simulink model "FourModesSerial"  (R2022b)
settings: Solver=FixedStepAuto  StartTime=0.0  StopTime=10.0  FixedStep=1e-3  RelTol=1e-3  EnableMultiTasking=on
undefined symbols (not defined in the file): D0, D1, D10, D11, D12, D13, D2, D3, D4, D5, D6, D7, D8, D9, PTA0, PTA1, PTA2, PTB23, PTB9, PTC16, PTC17, PTC2, PTC3, PTC4, PTD0, PTD1, PTD2, PTD3
libraries: frdmk64flib x17, etargetslib x2, dspstat3 x1
settings Model: ExtModeTrigDuration=5  Creator=16475  LastModifiedBy=16475
settings OptimizationCC: EnhancedBackFolding=on  PassReuseOutputArgsAs=Individual arguments  ZeroExternalMemoryAtStartup=off  ZeroInternalMemoryAtStartup=off  MaxStackSize=64  OptimizeBlockOrder=speed  DifferentSizesBufferReuse=on  OptimizationCustomize=off  EfficientTunableParamExpr=on
settings DebuggingCC: ParameterTunabilityLossMsg=error
settings HardwareCC: ProdBitPerPointer=32  ProdBitPerSizeT=32  ProdBitPerPtrDiffT=32  ProdLargestAtomicInteger=Long  ProdLargestAtomicFloat=Double  ProdWordSize=32  ProdHWDeviceType=ARM Compatible->ARM Cortex
settings SFSimCC: MATLABDynamicMemAlloc=off
settings RTWCC: Description=Embedded Coder  SystemTargetFile=ert.tlc  HardwareBoard=NXP FRDM-K64F  TLCOptions="-aInlineSetEventsForThisBaseRateFcn=TLC_FALSE -aSuppressMultiTaskScheduler=TLC_FALSE  -aRateBasedStepFcn=0"  TemplateMakefile=ert_default_tmf  Toolchain=GNU Tools for ARM Embedded Processors
settings CodeAppCC: ForceParamTrailComments=on  IgnoreCustomStorageClasses=off  OperatorAnnotations=on  SimulinkDataObjDesc=on  SFDataObjDesc=on  InsertBlockDesc=on
settings ERTTargetCC: ExtModeTransport=4  ExtModeMexFile=sendToCommService

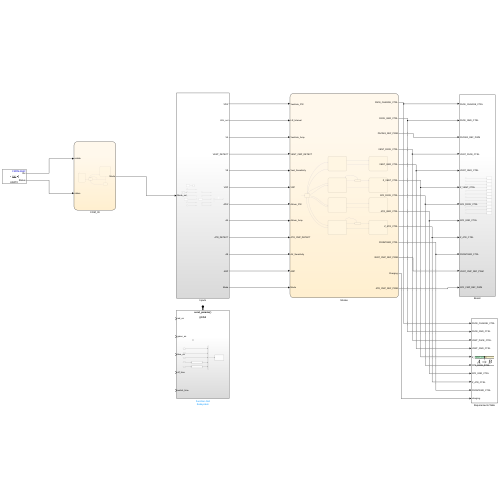
[thumbnail: Simulink's stored preview of the top-level diagram]
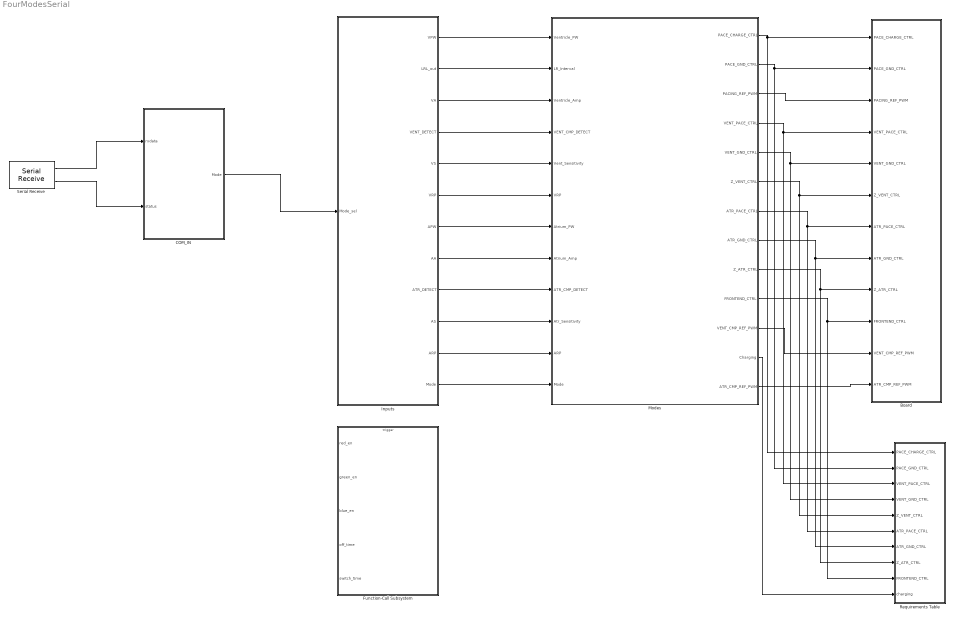
== system FourModesSerial ==
  Board : Subsystem
  COM_IN : Stateflow chart  TreatAsAtomicUnit=on
  Function-Call Subsystem : Subsystem  TreatAsAtomicUnit=on
  Inputs : Subsystem
  Modes : Stateflow chart  TreatAsAtomicUnit=on
      settings: PortSchema="{\"entries\":[{\"content\":{\"sides\":[{\"content\":{\"connectorIds\":[\"In1\",\"In2\",\"In3\",\"In4\",\"In5\",\"In6\",\"In7\",\"In8\",\"In9\",\"In10\",\"In11\",\"In12\"]},\"type\":\"ConnectorPlacement.EquallySpacedRectSide\",\"uuid\":\"a3e94f58-3093-42a5-91db-f56c9d127bee\"},{\"content\":{\"connectorIds\":[\"Out1\",\"Out2\",\"Out3\",\"Out5\",\"Out4\",\"Out7\",\"Out6\",\"Out8\",\"Out9\",\"Out10\",\"Out11\",\"Out12\",\"Out13\"],\"side\":\"RIGHT\"},\"type\":\"ConnectorPlacement.EquallySpacedRectSide\",\"uuid\":\"289ad049-9840-4721-af22-1385d5696f7c\"},{\"content\":{\"connectorIds\":[],\"side\":\"TOP\"},\"type\":\"ConnectorPlacement.EquallySpacedRectSide\",\"uuid\":\"4602f2ad-cb91-4c7a-9db6-6571445db01f\"}]},\"type\":\"ConnectorPlacement.EquallySpacedConnector\",\"uuid\":\"bfd50937-4990-4c1b-ba87-ff4dc7d3240f\"}],\"packageUris\":[\"http://schema.mathworks.com/mf0/Connector/R2020b\"],\"version\":\"1.0\"}"
  Requirements Table : Requirements Table  TreatAsAtomicUnit=on
  Serial Receive : frdmk64flib/Serial Receive  SCIModule=0  Baudrate=uint32(9600)  Parity=None  StopBits=1  HardwareFlowControl=None  ByteOrder=LittleEndian  DataType=uint8  DataLength=11  BlockingMode=off  OutputStatus=on  SampleTime=-1
  wires:
  Modes/11(VENT_CMP_REF_PWM) -> Board/11(VENT_CMP_REF_PWM)
  Modes/1(PACE_CHARGE_CTRL) -> Requirements Table/1(PACE_CHARGE_CTRL), Board/1(PACE_CHARGE_CTRL)
  Modes/2(PACE_GND_CTRL) -> Requirements Table/2(PACE_GND_CTRL), Board/2(PACE_GND_CTRL)
  Modes/3(PACING_REF_PWM) -> Board/3(PACING_REF_PWM)
  Modes/5(VENT_PACE_CTRL) -> Requirements Table/3(VENT_PACE_CTRL), Board/4(VENT_PACE_CTRL)
  Modes/4(VENT_GND_CTRL) -> Requirements Table/4(VENT_GND_CTRL), Board/5(VENT_GND_CTRL)
  Modes/7(Z_VENT_CTRL) -> Requirements Table/5(Z_VENT_CTRL), Board/6(Z_VENT_CTRL)
  Modes/6(ATR_PACE_CTRL) -> Requirements Table/6(ATR_PACE_CTRL), Board/7(ATR_PACE_CTRL)
  Modes/8(ATR_GND_CTRL) -> Requirements Table/7(ATR_GND_CTRL), Board/8(ATR_GND_CTRL)
  Modes/9(Z_ATR_CTRL) -> Requirements Table/8(Z_ATR_CTRL), Board/9(Z_ATR_CTRL)
  Modes/10(FRONTEND_CTRL) -> Requirements Table/9(FRONTEND_CTRL), Board/10(FRONTEND_CTRL)
  Modes/12(Charging) -> Requirements Table/10(charging)
  Inputs/1(VPW) -> Modes/1(Ventricle_PW)
  Inputs/2(LRL_out) -> Modes/2(LR_Interval)
  Inputs/3(VA) -> Modes/3(Ventricle_Amp)
  Inputs/4(VENT_DETECT) -> Modes/4(VENT_CMP_DETECT)
  Inputs/5(VS) -> Modes/5(Vent_Sensitivity)
  Inputs/6(VRP) -> Modes/6(VRP)
  Inputs/7(APW) -> Modes/7(Atrium_PW)
  Inputs/8(AA) -> Modes/8(Atrium_Amp)
  Inputs/9(ATR_DETECT) -> Modes/9(ATR_CMP_DETECT)
  Inputs/10(AS) -> Modes/10(Atr_Sensitivity)
  Inputs/11(ARP) -> Modes/11(ARP)
  Inputs/12(Mode) -> Modes/12(Mode)
  Modes/13(ATR_CMP_REF_PWM) -> Board/12(ATR_CMP_REF_PWM)
  Serial Receive/1 -> COM_IN/1(rxdata)
  Serial Receive/2 -> COM_IN/2(status)
  COM_IN/1(Mode) -> Inputs/1(Mode_sel)

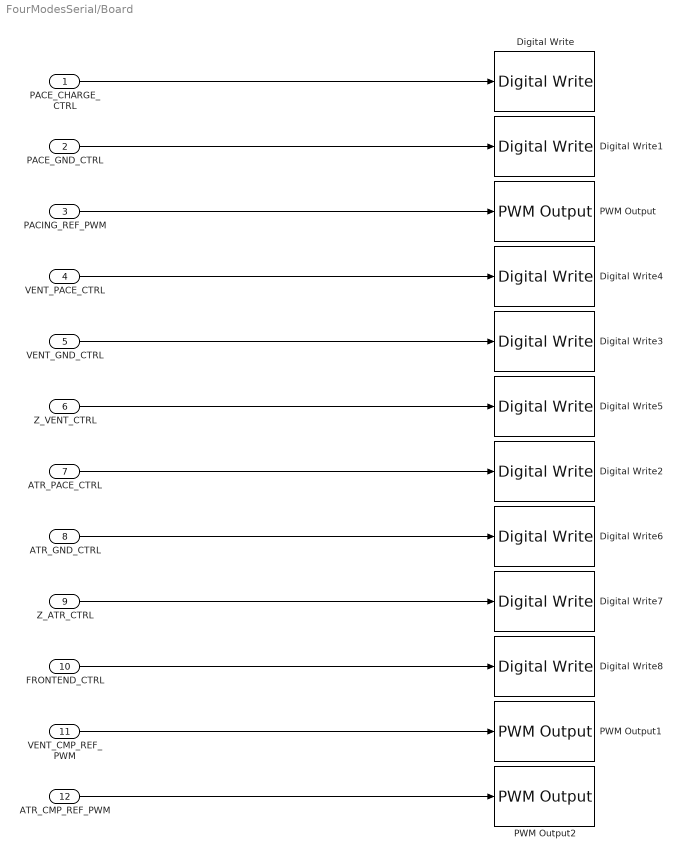
== system FourModesSerial/Board ==
  PACE_CHARGE_CTRL : Inport
  PACE_GND_CTRL : Inport  Port=2
  PACING_REF_PWM : Inport  Port=3
  VENT_PACE_CTRL : Inport  Port=4
  VENT_GND_CTRL : Inport  Port=5
  Z_VENT_CTRL : Inport  Port=6
  ATR_PACE_CTRL : Inport  Port=7
  ATR_GND_CTRL : Inport  Port=8
  Z_ATR_CTRL : Inport  Port=9
  FRONTEND_CTRL : Inport  Port=10
  VENT_CMP_REF_PWM : Inport  Port=11
  ATR_CMP_REF_PWM : Inport  Port=12
  Digital Write : frdmk64flib/Digital Write  Whichpin=PTB9 (D2)
  Digital Write1 : frdmk64flib/Digital Write  Whichpin=PTD0 (D10)
  Digital Write2 : frdmk64flib/Digital Write  Whichpin=PTA0 (D8)
  Digital Write3 : frdmk64flib/Digital Write  Whichpin=PTD3 (D12)
  Digital Write4 : frdmk64flib/Digital Write  Whichpin=PTC4 (D9)
  Digital Write5 : frdmk64flib/Digital Write  Whichpin=PTC3 (D7)
  Digital Write6 : frdmk64flib/Digital Write  Whichpin=PTD2 (D11)
  Digital Write7 : frdmk64flib/Digital Write  Whichpin=PTB23 (D4)
  Digital Write8 : frdmk64flib/Digital Write  Whichpin=PTD1 (D13)
  PWM Output : frdmk64flib/PWM Output  Whichpin=PTA2 (D5)  InitialFrequency=2000  InitialDutyCycle=0
  PWM Output1 : frdmk64flib/PWM Output  Whichpin=PTA1 (D3)  InitialFrequency=2000  InitialDutyCycle=0
  PWM Output2 : frdmk64flib/PWM Output  Whichpin=PTC2 (D6)  InitialFrequency=2000  InitialDutyCycle=0
  wires:
  Z_VENT_CTRL/1 -> Digital Write5/1
  VENT_GND_CTRL/1 -> Digital Write3/1
  PACE_CHARGE_CTRL/1 -> Digital Write/1
  PACE_GND_CTRL/1 -> Digital Write1/1
  VENT_PACE_CTRL/1 -> Digital Write4/1
  ATR_GND_CTRL/1 -> Digital Write6/1
  ATR_PACE_CTRL/1 -> Digital Write2/1
  PACING_REF_PWM/1 -> PWM Output/1
  Z_ATR_CTRL/1 -> Digital Write7/1
  FRONTEND_CTRL/1 -> Digital Write8/1
  VENT_CMP_REF_PWM/1 -> PWM Output1/1
  ATR_CMP_REF_PWM/1 -> PWM Output2/1

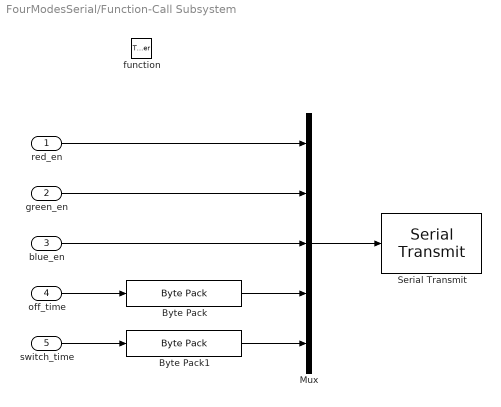
== system FourModesSerial/Function-Call Subsystem ==
  red_en : Inport
  green_en : Inport  Port=2
  blue_en : Inport  Port=3
  off_time : Inport  Port=4
  switch_time : Inport  Port=5
  function : TriggerPort  TriggerType=function-call  IsSimulinkFunction=on  FunctionName=send_params  VariantControl=(inherit)
  Byte Pack : etargetslib/Byte Pack  datatypes={'single'}  byteAlign=1
  Byte Pack1 : etargetslib/Byte Pack  datatypes={'uint16'}  byteAlign=1
  Mux : Mux  Inputs=5
  Serial Transmit : frdmk64flib/Serial Transmit  SCIModule=0  Baudrate=uint32(9600)  Parity=None  StopBits=1  HardwareFlowControl=None  ByteOrder=LittleEndian  BlockingMode=on  OutputStatus=off
  wires:
  off_time/1 -> Byte Pack/1
  switch_time/1 -> Byte Pack1/1
  Mux/1 -> Serial Transmit/1
  red_en/1 -> Mux/1
  green_en/1 -> Mux/2
  blue_en/1 -> Mux/3
  Byte Pack/1 -> Mux/4
  Byte Pack1/1 -> Mux/5

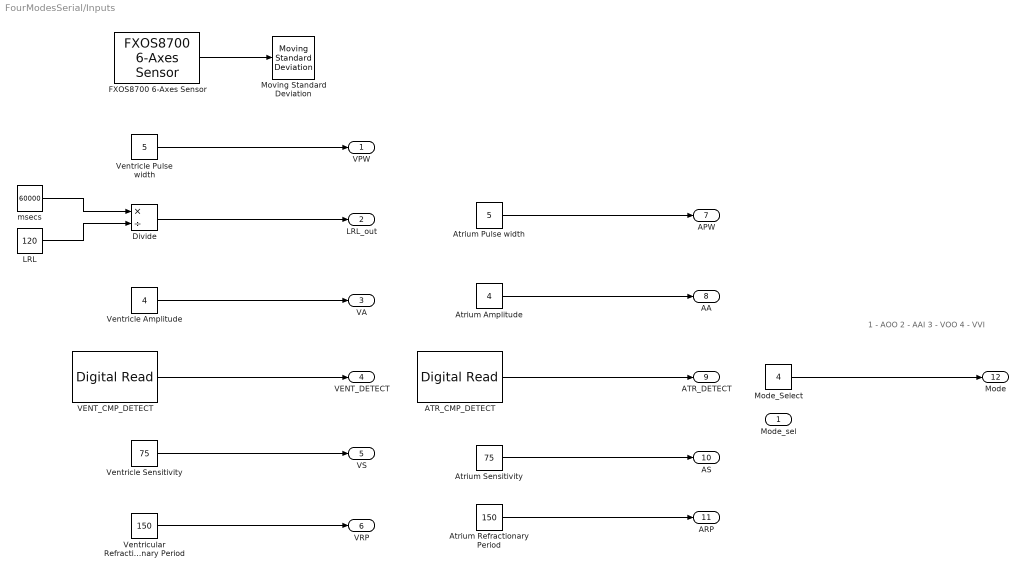
== system FourModesSerial/Inputs ==
  note: 1 - AOO
      | 2 - AAI
      | 3 - VOO
      | 4 - VVI
  Mode_sel : Inport
  ATR_CMP_DETECT : frdmk64flib/Digital Read  Whichpin=PTC16 (D0)  SampleTime=-1
  Atrium Amplitude : Constant  Value=4
  Atrium Pulse width : Constant  Value=5
  Atrium Refractionary Period : Constant  Value=150
  Atrium Sensitivity : Constant  Value=75
  Divide : Product  Inputs=*/
  FXOS8700 6-Axes Sensor : frdmk64flib/FXOS8700 6-Axes Sensor  Activesensor=Accelerometer only  ODR=800Hz  HybridODR=400Hz  Accelfullrange=-4g to +4g  SampleTime=-1
  LRL : Constant  Value=120
  Mode_Select : Constant  Value=4
  Moving Standard Deviation : dspstat3/Moving Standard Deviation  Method=Sliding window  ForgettingFactorPort=off  SpecifyWindowLength=on  WindowLength=4  OverlapLength=3  AllowArbitraryInputLength=off  ForgettingFactor=0.9  SimulateUsing=Code generation
  VENT_CMP_DETECT : frdmk64flib/Digital Read  Whichpin=PTC17 (D1)  SampleTime=-1
  Ventricle Amplitude : Constant  Value=4
  Ventricle Pulse width : Constant  Value=5
  Ventricle Sensitivity : Constant  Value=75
  Ventricular Refractionary Period : Constant  Value=150
  msecs : Constant  Value=60000
  VPW : Outport
  LRL_out : Outport  Port=2
  VA : Outport  Port=3
  VENT_DETECT : Outport  Port=4
  VS : Outport  Port=5
  VRP : Outport  Port=6
  APW : Outport  Port=7
  AA : Outport  Port=8
  ATR_DETECT : Outport  Port=9
  AS : Outport  Port=10
  ARP : Outport  Port=11
  Mode : Outport  Port=12
  wires:
  Ventricle Pulse width/1 -> VPW/1
  Divide/1 -> LRL_out/1
  msecs/1 -> Divide/1
  LRL/1 -> Divide/2
  Ventricle Amplitude/1 -> VA/1
  VENT_CMP_DETECT/1 -> VENT_DETECT/1
  Ventricle Sensitivity/1 -> VS/1
  Ventricular Refractionary Period/1 -> VRP/1
  ATR_CMP_DETECT/1 -> ATR_DETECT/1
  Atrium Pulse width/1 -> APW/1
  Atrium Amplitude/1 -> AA/1
  Atrium Sensitivity/1 -> AS/1
  Atrium Refractionary Period/1 -> ARP/1
  Mode_Select/1 -> Mode/1
  FXOS8700 6-Axes Sensor/1 -> Moving Standard Deviation/1

== stateflow chart FourModesSerial/Modes ==
  state Charging_AOO
    entry:
    ATR_PACE_CTRL = false;
    VENT_PACE_CTRL = false;
    PACING_REF_PWM = ((Atrium_Amp/5)*100);
    PACE_CHARGE_CTRL = true;
    PACE_GND_CTRL = true;
    Z_ATR_CTRL = false;
    Z_VENT_CTRL = false;
    ATR_GND_CTRL = true;
    VENT_GND_CTRL = false;
    Charging = true;
  state Discharging_AOO
    entry:
    PACE_CHARGE_CTRL = false;
    PACE_GND_CTRL = true;
    ATR_PACE_CTRL = true;
    VENT_PACE_CTRL = false;
    Z_ATR_CTRL = false;
    Z_VENT_CTRL = false;
    ATR_GND_CTRL = false;
    VENT_GND_CTRL = false;
    Charging = false;
  state Charging_AAI
    entry:
    ATR_PACE_CTRL = false;
    VENT_PACE_CTRL = false;
    PACING_REF_PWM = ((Atrium_Amp/5)*100);
    PACE_CHARGE_CTRL = true;
    PACE_GND_CTRL = true;
    Z_ATR_CTRL = false;
    Z_VENT_CTRL = false;
    ATR_GND_CTRL = true;
    VENT_GND_CTRL = false;
    FRONTEND_CTRL = true;
    ATR_CMP_REF_PWM = Atr_Sensitivity;
    Charging = true;
  state Discharging_AAI
    entry:
    PACE_CHARGE_CTRL = false;
    PACE_GND_CTRL = true;
    ATR_PACE_CTRL = true;
    VENT_PACE_CTRL = false;
    Z_ATR_CTRL = false;
    Z_VENT_CTRL = false;
    ATR_GND_CTRL = false;
    VENT_GND_CTRL = false;
    FRONTEND_CTRL = false;
    Charging = false;
  state Check_State_AAI
  state Init
  state Charging_VOO
    entry:
    ATR_PACE_CTRL = false;
    VENT_PACE_CTRL = false;
    PACING_REF_PWM = ((Ventricle_Amp/5)*100);
    PACE_CHARGE_CTRL = true;
    PACE_GND_CTRL = true;
    Z_ATR_CTRL = false;
    Z_VENT_CTRL = false;
    ATR_GND_CTRL = false;
    VENT_GND_CTRL = true;
    Charging = true;
  state Discharging_VOO
    entry:
    PACE_CHARGE_CTRL = false;
    PACE_GND_CTRL = true;
    ATR_PACE_CTRL = false;
    VENT_PACE_CTRL = true;
    Z_ATR_CTRL = false;
    Z_VENT_CTRL = false;
    ATR_GND_CTRL = false;
    VENT_GND_CTRL = false;
    Charging = false;
  state Charging_Sensing_VVI
    entry:
    ATR_PACE_CTRL = false;
    VENT_PACE_CTRL = false;
    PACING_REF_PWM = ((Ventricle_Amp/5)*100);
    PACE_CHARGE_CTRL = true;
    PACE_GND_CTRL = true;
    Z_ATR_CTRL = false;
    Z_VENT_CTRL = false;
    ATR_GND_CTRL = false;
    VENT_GND_CTRL = true;
    FRONTEND_CTRL = true;
    VENT_CMP_REF_PWM = Vent_Sensitivity;
    Charging = true;
  state Discharging_VVI
    entry:
    PACE_CHARGE_CTRL = false;
    PACE_GND_CTRL = true;
    ATR_PACE_CTRL = false;
    VENT_PACE_CTRL = true;
    Z_ATR_CTRL = false;
    Z_VENT_CTRL = false;
    ATR_GND_CTRL = false;
    VENT_GND_CTRL = false;
    FRONTEND_CTRL = false;
    Charging = false;
  state Check_State_VVI
  Charging_AOO -> Discharging_AOO [order 1] : [after(LR_Interval - Atrium_PW,msec)]
  Init -> Charging_AOO [order 1] : [Mode == 1]
  Discharging_AOO -> Charging_AOO : [after(Atrium_PW,msec)]
  Charging_AOO -> Init [order 2] : [Mode ~= 1]
  Check_State_AAI -> Charging_AAI [order 1] : [ATR_CMP_DETECT == true]
  Charging_AAI -> Check_State_AAI [order 1] : [after(ARP,msec)]
  Check_State_AAI -> Discharging_AAI [order 2] : [after(LR_Interval - ARP,msec)]
  Charging_AAI -> Init [order 2] : [Mode ~= 2]
  Init -> Charging_AAI [order 2] : [Mode == 2]
  Discharging_AAI -> Charging_AAI : [after(Atrium_PW,msec)]
  (default) -> Init
  Init -> Charging_VOO [order 3] : [Mode == 3]
  Charging_VOO -> Init [order 2] : [Mode ~= 3]
  Charging_Sensing_VVI -> Init [order 2] : [Mode ~= 4]
  Init -> Charging_Sensing_VVI [order 4] : [Mode == 4]
  Charging_VOO -> Discharging_VOO [order 1] : [after(LR_Interval - Ventricle_PW,msec)]
  Discharging_VOO -> Charging_VOO : [after(Ventricle_PW,msec)]
  Check_State_VVI -> Charging_Sensing_VVI [order 1] : [VENT_CMP_DETECT == true]
  Check_State_VVI -> Discharging_VVI [order 2] : [after(LR_Interval - VRP,msec)]
  Charging_Sensing_VVI -> Check_State_VVI [order 1] : [after(VRP,msec)]
  Discharging_VVI -> Charging_Sensing_VVI : [after(Ventricle_PW,msec)]
  data: Ventricle_PW input double; LR_Interval input double; PACE_CHARGE_CTRL output boolean; PACE_GND_CTRL output boolean; PACING_REF_PWM output double; VENT_GND_CTRL output boolean; VENT_PACE_CTRL output boolean; ATR_PACE_CTRL output boolean; Z_VENT_CTRL output boolean; Ventricle_Amp input double; ATR_GND_CTRL output boolean; Z_ATR_CTRL output boolean; VENT_CMP_DETECT input boolean; FRONTEND_CTRL output boolean; VENT_CMP_REF_PWM output double; Vent_Sensitivity input double; VRP input double; Charging output; Atrium_PW input; Atrium_Amp input; ATR_CMP_DETECT input; Atr_Sensitivity input; ARP input; Mode input; ATR_CMP_REF_PWM output

== stateflow chart FourModesSerial/Requirements Table ==
  (default) -> (junction 1073742466)
  (junction 1073742466) -> (junction 1073742467) : {
      | % SF_REQ_REV_07
      | }
  (junction 1073742467) -> (junction 1073742469) : {
      | % HEADER_ASSIGNMENTS
      |
      | }
  (junction 1073742469) -> (junction 1073742471) : {
      | % START_A_4
      | }
  (junction 1073742471) -> (junction 1073742473) : {
      | }
  (junction 1073742473) -> (junction 1073742475)
  (junction 1073742475) -> (junction 1073742477) : {
      | }
  (junction 1073742477) -> (junction 1073742479) : {
      | % END_A_4
      | }
  (junction 1073742479) -> (junction 1073742481) : {
      | % START_R_1
      | }
  (junction 1073742481) -> (junction 1073742483) : {
      | }
  (junction 1073742483) -> (junction 1073742485)
  (junction 1073742485) -> (junction 1073742487) [order 1] : [(((prev(charging)) == (prev(charging) == false)))]
  (junction 1073742485) -> (junction 1073742493) [order 2]
  (junction 1073742487) -> (junction 1073742489) : {
      | reqtable_postcondition((((PACE_CHARGE_CTRL) == (true))) && (((PACE_GND_CTRL) == (true))) && (((VENT_PACE_CTRL) == (false))) && (((VENT_GND_CTRL) == (true))) && (((Z_VENT_CTRL) == (false))) && (((ATR_PACE_CTRL) == (false))) && (((ATR_GND_CTRL) == (false))) && (((Z_ATR_CTRL) == (false))) && (((FRONTEND_CTRL) == (true))) && (((charging) == (true))), 'R:1');
      |
      |
      | }
  (junction 1073742489) -> (junction 1073742491) : {
      | }
  (junction 1073742491) -> (junction 1073742493)
  (junction 1073742493) -> (junction 1073742495)
  (junction 1073742495) -> (junction 1073742497) : {
      | % END_R_1
      | }
  (junction 1073742497) -> (junction 1073742499) : {
      | % START_R_7
      | }
  (junction 1073742499) -> (junction 1073742501) : {
      | }
  (junction 1073742501) -> (junction 1073742503)
  (junction 1073742503) -> (junction 1073742505) [order 1] : [(((prev(charging)) == (prev(charging) == true)))]
  (junction 1073742503) -> (junction 1073742511) [order 2]
  (junction 1073742505) -> (junction 1073742507) : {
      | reqtable_postcondition((((PACE_CHARGE_CTRL) == (false))) && (((PACE_GND_CTRL) == (true))) && (((VENT_PACE_CTRL) == (true))) && (((VENT_GND_CTRL) == (false))) && (((Z_VENT_CTRL) == (false))) && (((ATR_PACE_CTRL) == (false))) && (((ATR_GND_CTRL) == (false))) && (((Z_ATR_CTRL) == (false))) && (((FRONTEND_CTRL) == (false))) && (((charging) == (false))), 'R:2');
      |
      |
      | }
  (junction 1073742507) -> (junction 1073742509) : {
      | }
  (junction 1073742509) -> (junction 1073742511)
  (junction 1073742511) -> (junction 1073742513)
  (junction 1073742513) -> (junction 1073742515) : {
      | % END_R_7
      | }
  data: PACE_CHARGE_CTRL input boolean; PACE_GND_CTRL input boolean; VENT_PACE_CTRL input boolean; VENT_GND_CTRL input boolean; Z_VENT_CTRL input boolean; ATR_PACE_CTRL input boolean; ATR_GND_CTRL input boolean; Z_ATR_CTRL input boolean; FRONTEND_CTRL input boolean; charging input boolean

== stateflow chart FourModesSerial/COM_IN ==
  state SET_PARAM
    % Still need to adapt to fit our model
    entry:
    Mode = rxdata(3);
    green_en =  rxdata(4);
    blue_en = rxdata(5);
    off_time = typecast(rxdata(6:9), 'single');
    switch_time = typecast(rxdata(10:11), 'uint16');
  state Init
    entry:
    mode = 1;
    Ventricular_Pulse_Width = 5;
    LRL = 120;
    Ventricular_Amplitude = 4;
    Ventricle_Sensitivity = 75;
    VRP = 150;
    Atrium_Pulse_Width = 5;
    Atrium_Amplitude = 4;
    Atrium_Sensitivity = 2.3;
    ARP = 150;
  state Standby
    %wait for COM
  state ECHO_PARAM
    entry:
    send_params();
  (default) -> Init
  SET_PARAM -> Standby
  (junction 59) -> SET_PARAM [order 2] : [rxdata(2)==hex2dec('55')]
  (junction 65) -> Standby [order 2]
  Init -> Standby
  Standby -> (junction 65) : [status == 0]
  (junction 65) -> (junction 59) [order 1] : [rxdata(1)==hex2dec('16')]
  (junction 59) -> ECHO_PARAM [order 1] : [rxdata(2)==hex2dec('22')]
  ECHO_PARAM -> Standby
  data: rxdata input; status input; Mode output
